simulink library "INP_BRK_EB"  (R2023b)
settings: Solver=VariableStepAuto  StartTime=0.0  StopTime=10.0  RelTol=1e-3
settings Model: Creator=blatak  LastModifiedBy=blatak

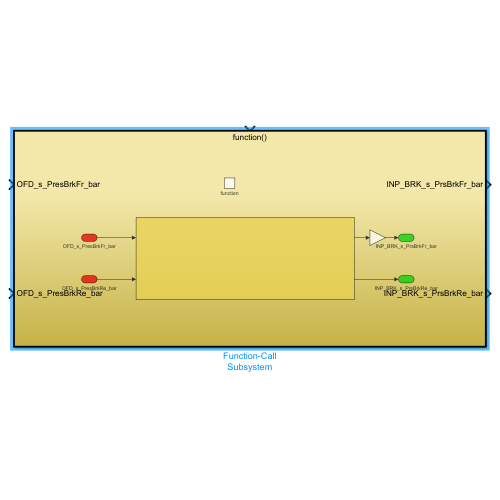
[thumbnail: Simulink's stored preview of the top-level diagram]
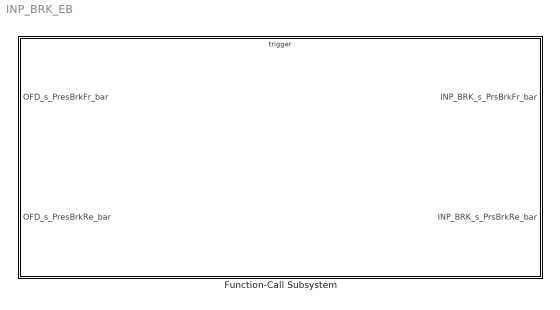
== system INP_BRK_EB ==
  Function-Call Subsystem : Subsystem  TreatAsAtomicUnit=on

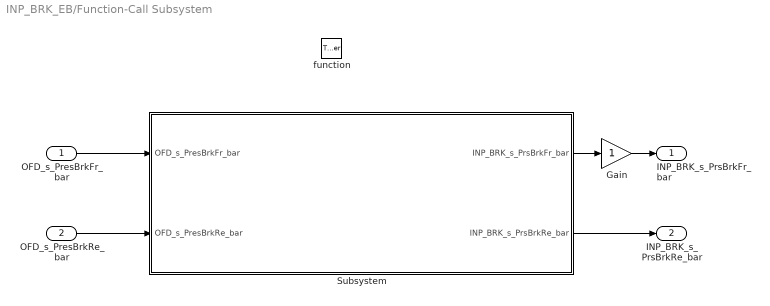
== system INP_BRK_EB/Function-Call Subsystem ==
  OFD_s_PresBrkFr_bar : Inport
  OFD_s_PresBrkRe_bar : Inport  Port=2
  function : TriggerPort  TriggerType=function-call  VariantControl=(inherit)
  Gain : Gain
  Subsystem : Subsystem
  INP_BRK_s_PrsBrkFr_bar : Outport
  INP_BRK_s_PrsBrkRe_bar : Outport  Port=2
  wires:
  Subsystem/2(INP_BRK_s_PrsBrkRe_bar) -> INP_BRK_s_PrsBrkRe_bar/1
  Subsystem/1(INP_BRK_s_PrsBrkFr_bar) -> Gain/1
  OFD_s_PresBrkFr_bar/1 -> Subsystem/1(OFD_s_PresBrkFr_bar)
  OFD_s_PresBrkRe_bar/1 -> Subsystem/2(OFD_s_PresBrkRe_bar)
  Gain/1 -> INP_BRK_s_PrsBrkFr_bar/1

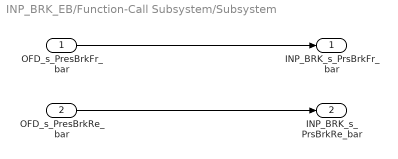
== system INP_BRK_EB/Function-Call Subsystem/Subsystem ==
  OFD_s_PresBrkFr_bar : Inport
  OFD_s_PresBrkRe_bar : Inport  Port=2
  INP_BRK_s_PrsBrkFr_bar : Outport
  INP_BRK_s_PrsBrkRe_bar : Outport  Port=2
  wires:
  OFD_s_PresBrkRe_bar/1 -> INP_BRK_s_PrsBrkRe_bar/1
  OFD_s_PresBrkFr_bar/1 -> INP_BRK_s_PrsBrkFr_bar/1
